simulink model "AMCLIB_TrackObsrv_BAM_F32"  (Simulink 8.3)
settings: Solver=ode45  StartTime=0.0  StopTime=10.0  RelTol=1e-3
undefined symbols (not defined in the file): f32C1, f32CC1sc, f32CC2sc, u16IntegNShift, u16NShift
settings Model: Creator=RE004C  LastModifiedBy=RE004C
settings DataIOCC: SignalLoggingSaveFormat=Dataset
settings DebuggingCC: UnderspecifiedInitializationDetection=Simplified  StateNameClashWarn=none
settings GRTTargetCC: CombineOutputUpdateFcns=on  GRTInterface=off

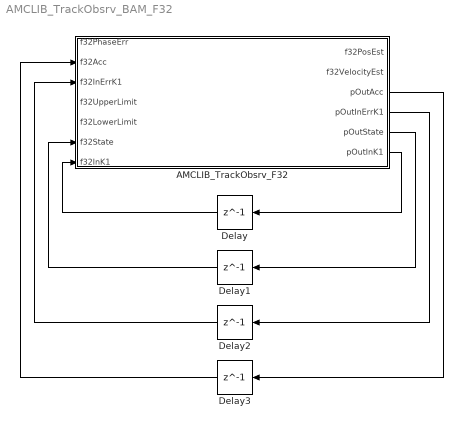
== system AMCLIB_TrackObsrv_BAM_F32 ==
  AMCLIB_TrackObsrv_F32 : Subsystem  mask(AMCLIB_TrackObsrv_F32){f32CC1sc=f32CC1sc, f32CC2sc=f32CC2sc, u16NShift=u16NShift, f32C1=f32C1, u16IntegNShift=u16IntegNShift}
      mask help: Bit accurate model of the tracking observer function.
      mask init:
      | pos = get_param(gcb, 'Position');width = pos(3) - pos(1); height = pos(4) - pos(2);tX=width/2;tY=height*0.9;
      mask Display: color('black');port_label('input',1,'f32PhaseErr');port_label('input',2,'f32Acc');port_label('input',3,'f32InErrK1');port_label('input',4,'f32UpperLimit');port_label('input',5,'f32LowerLimit');port_label('input',6,'f32State');port_label('input',7,'f32InK1');port_label('output',1,'f32PosEst');port_label('output',2,'f32VelocityEst');port_label('output',3,'pOutAcc');port_label('output',4,'pOutInErrK1');port_label('output',5,'pOutState');port_label('output',6,'pOutInK1');color('black');disp('AMCLIB_TrackObsrv_F32');color('blue');text(tX,tY, 'BAM', 'horizontalAlignment', 'center');
  Delay{,1..3} (4 alike) : Delay  DelayLength=1  InitialCondition=0
  wires:
  AMCLIB_TrackObsrv_F32/6(pOutInK1) -> Delay/1
  Delay/1 -> AMCLIB_TrackObsrv_F32/7(f32InK1)
  AMCLIB_TrackObsrv_F32/5(pOutState) -> Delay1/1
  Delay1/1 -> AMCLIB_TrackObsrv_F32/6(f32State)
  AMCLIB_TrackObsrv_F32/4(pOutInErrK1) -> Delay2/1
  Delay2/1 -> AMCLIB_TrackObsrv_F32/3(f32InErrK1)
  AMCLIB_TrackObsrv_F32/3(pOutAcc) -> Delay3/1
  Delay3/1 -> AMCLIB_TrackObsrv_F32/2(f32Acc)

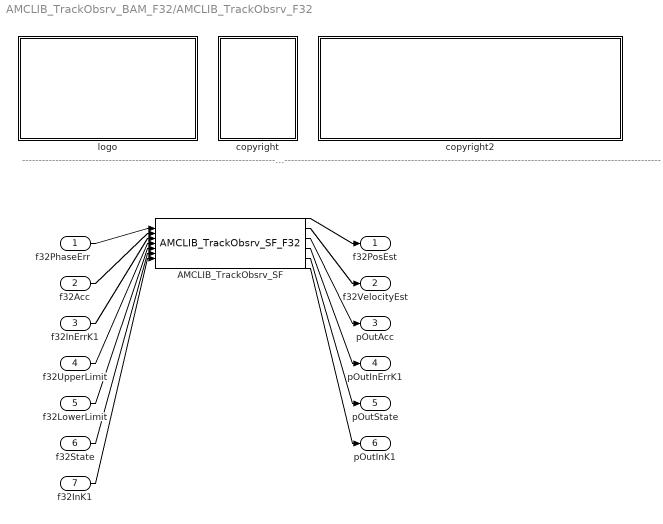
== system AMCLIB_TrackObsrv_BAM_F32/AMCLIB_TrackObsrv_F32 ==
  note: ---------------------------------------------------------------------------------------------------------------------------------------------------------------------------------------------------
  f32PhaseErr : Inport
  f32Acc : Inport  Port=2
  f32InErrK1 : Inport  Port=3
  f32UpperLimit : Inport  Port=4
  f32LowerLimit : Inport  Port=5
  f32State : Inport  Port=6
  f32InK1 : Inport  Port=7
  AMCLIB_TrackObsrv_SF : S-Function  FunctionName=AMCLIB_TrackObsrv_SF_F32  Parameters=f32CC1sc,f32CC2sc,u16NShift,f32C1,u16IntegNShift  EnableBusSupport=off
  copyright : Subsystem
      mask Display: text(10,90,'FILE:');text(10,75,'DESRIPTION:');text(10,60,'COPYRIGHT:');text(10,45,'VERSION:');text(10,30,'DATE:')
  copyright2 : Subsystem
      mask Display: text(10,90,'AMCLIB_TrackObsrv_BAM_F32.mdl');text(10,75,'Tracking observer function.');text(10,60,'NXP');text(10,45,'1.0');text(10,30,'29-Jul-2016');
  logo : Subsystem
      mask Display: image(imread('logo.jpg'))
  f32PosEst : Outport
  f32VelocityEst : Outport  Port=2
  pOutAcc : Outport  Port=3
  pOutInErrK1 : Outport  Port=4
  pOutState : Outport  Port=5
  pOutInK1 : Outport  Port=6
  wires:
  f32PhaseErr/1 -> AMCLIB_TrackObsrv_SF/1
  f32Acc/1 -> AMCLIB_TrackObsrv_SF/2
  f32InErrK1/1 -> AMCLIB_TrackObsrv_SF/3
  f32UpperLimit/1 -> AMCLIB_TrackObsrv_SF/4
  f32LowerLimit/1 -> AMCLIB_TrackObsrv_SF/5
  f32State/1 -> AMCLIB_TrackObsrv_SF/6
  f32InK1/1 -> AMCLIB_TrackObsrv_SF/7
  AMCLIB_TrackObsrv_SF/1 -> f32PosEst/1
  AMCLIB_TrackObsrv_SF/2 -> f32VelocityEst/1
  AMCLIB_TrackObsrv_SF/3 -> pOutAcc/1
  AMCLIB_TrackObsrv_SF/4 -> pOutInErrK1/1
  AMCLIB_TrackObsrv_SF/5 -> pOutState/1
  AMCLIB_TrackObsrv_SF/6 -> pOutInK1/1

== system AMCLIB_TrackObsrv_BAM_F32/AMCLIB_TrackObsrv_F32/copyright ==

== system AMCLIB_TrackObsrv_BAM_F32/AMCLIB_TrackObsrv_F32/copyright2 ==

== system AMCLIB_TrackObsrv_BAM_F32/AMCLIB_TrackObsrv_F32/logo ==
